simulink model "lab3es1"  (R2021a)
settings: Solver=VariableStepAuto  StartTime=0.0  StopTime=30  RelTol=1e-3
values from neighbouring files (symbols this model uses):
  b = 1.0    (= 1)    [VarLab3.m]
  g = 9.8    [VarLab3.m]
  Ie = I+m*l^2    (= 0.026047)    [VarLab3.m]
  k = 10    [VarLab3.m]
  K = [-0.02, -1.1, 7.5, 0.7]    [VarLab3.m]
  l = 0.305    [VarLab3.m]
  m = 0.21    [VarLab3.m]
  Me = m+M    (= 0.665)    [VarLab3.m]
  x = [0, 0, pi/8, 0]    [VarLab3.m]
settings Model: Creator=bonvoltnuovo  LastModifiedBy=bonvoltnuovo

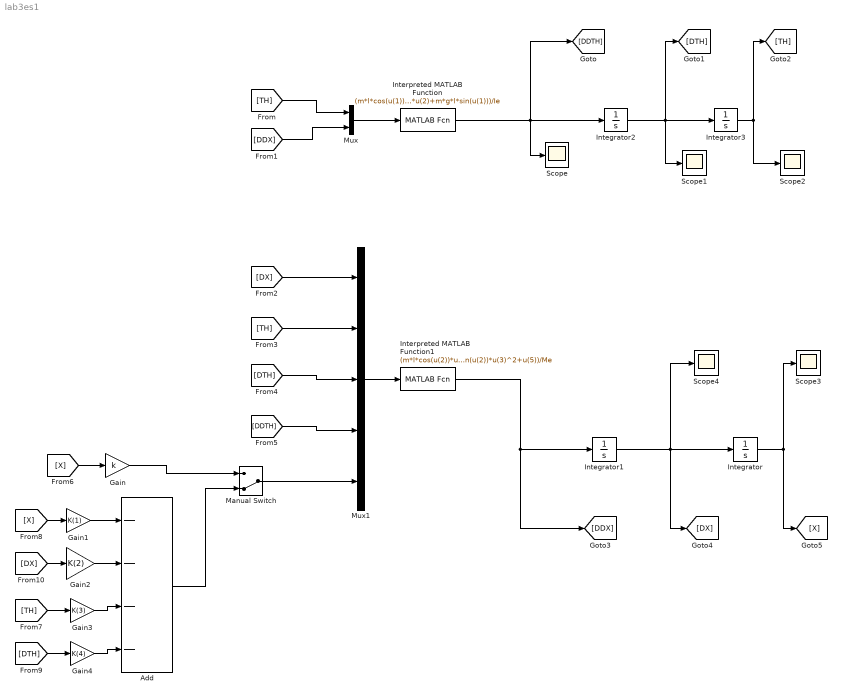
== system lab3es1 ==
  Add : Sum  Inputs=----
  Gain : Gain  Gain=k
  Gain1 : Gain  Gain=K(1)
  Gain2 : Gain  Gain=K(2)
  Gain3 : Gain  Gain=K(3)
  Gain4 : Gain  Gain=K(4)
  Integrator : Integrator  InitialCondition=x(1)
  Integrator1 : Integrator  InitialCondition=x(2)
  Integrator2 : Integrator  InitialCondition=x(4)
  Integrator3 : Integrator  InitialCondition=x(3)
  Interpreted MATLAB Function : MATLABFcn  MATLABFcn=(m*l*cos(u(1))*u(2)+m*g*l*sin(u(1)))/Ie
  Interpreted MATLAB Function1 : MATLABFcn  MATLABFcn=(m*l*cos(u(2))*u(4)-b*u(1)-m*l*sin(u(2))*u(3)^2+u(5))/Me
  Manual Switch : ManualSwitch  CurrentSetting=0
  Mux : Mux  Inputs=2
  Mux1 : Mux  Inputs=5
  Scope{,1..4} (5 alike) : Scope
  wires:
  [DDX] -> Mux/2
  Mux/1 -> Interpreted MATLAB Function/1
  [TH] -> Mux/1
  Integrator2/1 -> Scope1/1, Integrator3/1, [DTH]
  Integrator3/1 -> Scope2/1, [TH]
  Integrator/1 -> [X], Scope3/1
  Integrator1/1 -> Scope4/1, Integrator/1, [DX]
  Interpreted MATLAB Function/1 -> Scope/1, [DDTH], Integrator2/1
  [DDTH] -> Mux1/4
  [TH] -> Mux1/2
  [DTH] -> Mux1/3
  [DX] -> Mux1/1
  Interpreted MATLAB Function1/1 -> Integrator1/1, [DDX]
  Mux1/1 -> Interpreted MATLAB Function1/1
  [X] -> Gain/1
  Gain/1 -> Manual Switch/1
  Manual Switch/1 -> Mux1/5
  [X] -> Gain1/1
  [DX] -> Gain2/1
  [TH] -> Gain3/1
  [DTH] -> Gain4/1
  Gain4/1 -> Add/4
  Gain3/1 -> Add/3
  Gain2/1 -> Add/2
  Gain1/1 -> Add/1
  Add/1 -> Manual Switch/2
